simulink model "aaaa"  (R2020b)
settings: Solver=VariableStepAuto  StartTime=0.0  StopTime=10.0  RelTol=1e-3
undefined symbols (not defined in the file): DiscIntNeverNeededParam
settings Model: SimSIMDOptimization=Portable  Creator=aminamid  LastModifiedBy=aminamid

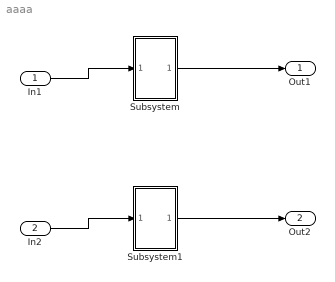
== system aaaa ==
  In1 : Inport
  In2 : Inport  Port=2
  Subsystem : Subsystem
  Subsystem1 : Subsystem
  Out1 : Outport
  Out2 : Outport  Port=2
  wires:
  In1/1 -> Subsystem/1(In1)
  Subsystem/1(Out1) -> Out1/1
  Subsystem1/1(Out1) -> Out2/1
  In2/1 -> Subsystem1/1(In1)

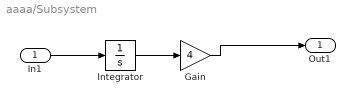
== system aaaa/Subsystem ==
  In1 : Inport
  Gain : Gain  Gain=4
  Integrator : Integrator
  Out1 : Outport
  wires:
  Integrator/1 -> Gain/1
  In1/1 -> Integrator/1
  Gain/1 -> Out1/1

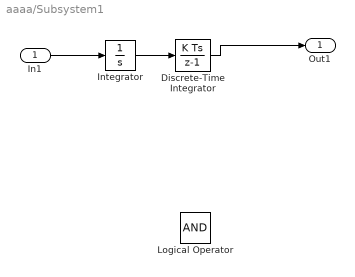
== system aaaa/Subsystem1 ==
  In1 : Inport
  Discrete-Time Integrator : DiscreteIntegrator  SampleTime=-1  ICPrevOutput=DiscIntNeverNeededParam  ICPrevScaledInput=DiscIntNeverNeededParam
  Integrator : Integrator
  Logical Operator : Logic  AllPortsSameDT=off  OutDataTypeStr=boolean
  Out1 : Outport
  wires:
  In1/1 -> Integrator/1
  Integrator/1 -> Discrete-Time Integrator/1
  Discrete-Time Integrator/1 -> Out1/1
